simulink model "mbed_nucleo_f303_max11300"  (R2015a)
settings: Solver=ode45  StartTime=0.0  StopTime=10.0  RelTol=1e-3
undefined symbols (not defined in the file or in its folder): Ended, Single
libraries: mbed_lib x10, simulink x2, mbed_targets_stm_disco_f407 x2, mbed_targets_stm_nucleo_f303 x1
settings Model: Creator=Stuv  LastModifiedBy=Stuv

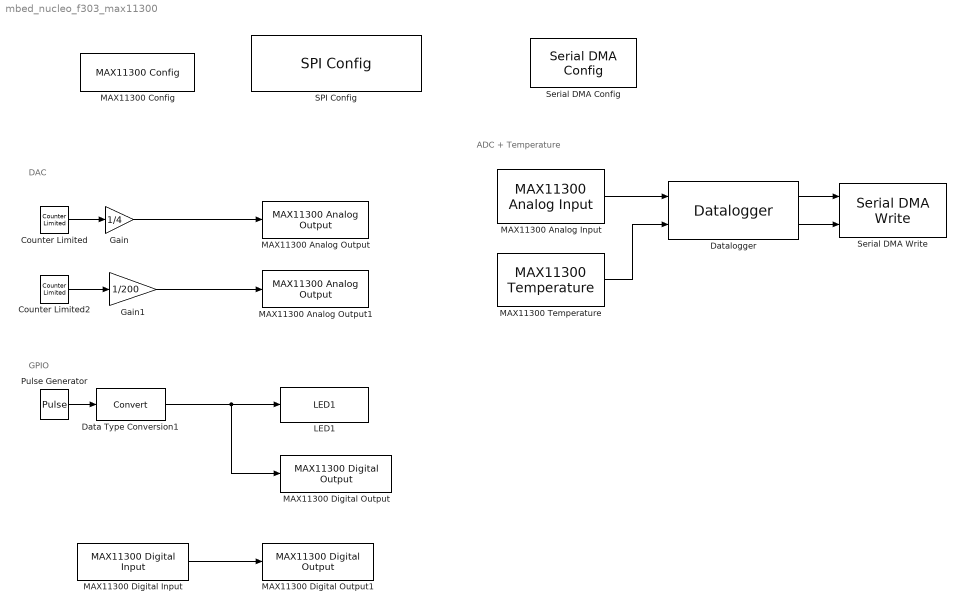
== system mbed_nucleo_f303_max11300 ==
  note: ADC + Temperature
  note: GPIO
  note: DAC
  Counter Limited : simulink/Sources/Counter Limited  uplimit=4  tsamp=-1
  Counter Limited2 : simulink/Sources/Counter Limited  uplimit=100  tsamp=-1
  Data Type Conversion1 : DataTypeConversion
  Datalogger : mbed_lib/Utilities/Datalogger  TypeInputPorts={ 'single' 1 'single' 1 }  TypeOfInputs={'1*single','1*single'}  BufferSize=40  errEn=off  SampleTime=-1
  Gain : Gain  Gain=1/4  OutDataTypeStr=single
  Gain1 : Gain  Gain=1/200  OutDataTypeStr=single
  LED1 : mbed_targets_stm_nucleo_f303/LED1  Parameter1=0
  MAX11300 Analog Input : mbed_lib/SPI/MAX11300 Analog Input  CsPort=B  CsPin=1  InputType=Single-Ended  Mode=relative  PosPin=0  NegPin=0  Power=1  Range=-5 to +5  Ref=Internal (2.5 V)
  MAX11300 Analog Output : mbed_lib/SPI/MAX11300 Analog Output  CsPort=B  CsPin=1  Pin=1  Mode=relative  Range=0 to +10 V
  MAX11300 Analog Output1 : mbed_lib/SPI/MAX11300 Analog Output  CsPort=B  CsPin=1  Pin=5  Mode=relative  Range=0 to +10 V
  MAX11300 Config : mbed_lib/SPI/MAX11300 Config  Priority=1  SpiPort=1  CsPort=B  CsPin=1  AdcRate=400 kSPS  DacRef=Internal (2.5 V)  TempCh0=on  TempCh1=off  TempCh2=off
  MAX11300 Digital Input : mbed_lib/SPI/MAX11300 Digital Input  CsPort=B  CsPin=1  Pin=2  Thresh=2048
  MAX11300 Digital Output : mbed_lib/SPI/MAX11300 Digital Output  CsPort=B  CsPin=1  Pin=3  Level=2^12-1
  MAX11300 Digital Output1 : mbed_lib/SPI/MAX11300 Digital Output  CsPort=B  CsPin=1  Pin=4  Level=2^11
  MAX11300 Temperature : mbed_lib/SPI/MAX11300 Temperature  CsPort=B  CsPin=1  Channel=Internal
  Pulse Generator : DiscretePulseGenerator  PulseType=Time based  PulseWidth=50
  SPI Config : mbed_lib/SPI/SPI Config  Priority=0  SpiPort=1  SParameter6=1000000  SParameter2=B  SParameter3=15  SParameter4=B  SParameter5=14  SCK_PORT=B  SCK_PIN=13
  Serial DMA Config : mbed_targets_stm_disco_f407/Serial DMA Config  SerialPort=2  TxPort=A  TxPin=2  RxPort=A  RxPin=3  BaudRate=115200
  Serial DMA Write : mbed_targets_stm_disco_f407/Serial DMA Write  SerialPort=2  numData=on  SampleTime=-1
  wires:
  Datalogger/1 -> Serial DMA Write/1
  Datalogger/2 -> Serial DMA Write/2
  MAX11300 Temperature/1 -> Datalogger/2
  Pulse Generator/1 -> Data Type Conversion1/1
  Data Type Conversion1/1 -> LED1/1, MAX11300 Digital Output/1
  MAX11300 Digital Input/1 -> MAX11300 Digital Output1/1
  Counter Limited/1 -> Gain/1
  Gain/1 -> MAX11300 Analog Output/1
  Counter Limited2/1 -> Gain1/1
  Gain1/1 -> MAX11300 Analog Output1/1
  MAX11300 Analog Input/1 -> Datalogger/1
